simulink model "GNN_11612319_Ajay"  (R2021a)
settings: Solver=VariableStepAuto  StartTime=0.0  StopTime=1.0  RelTol=1e-8  AbsTol=1e-8
InitFcn:
  | I=eye(2);
  | k=10;
undefined symbols (not defined in the file): m
libraries: neural x1
settings Model: Creator=Mannaiyar  LastModifiedBy=Mannaiyar

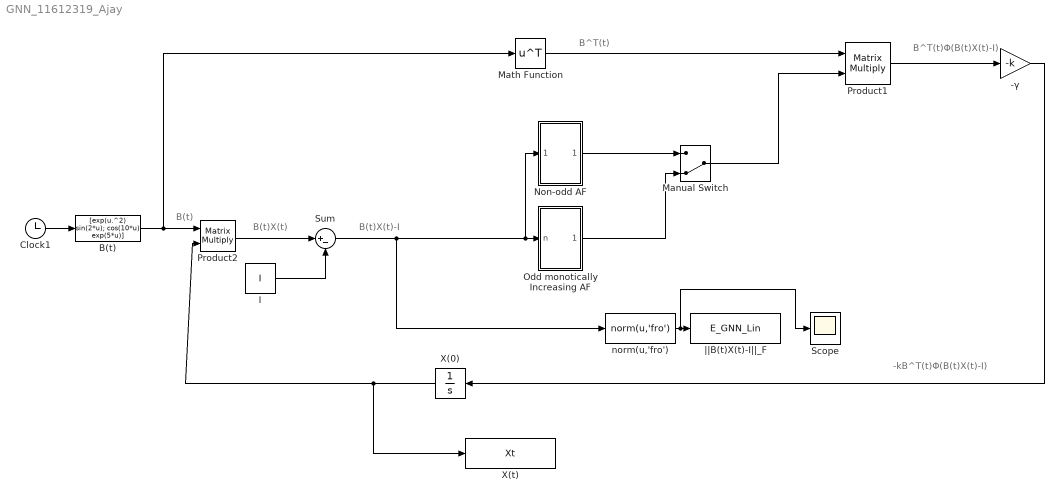
== system GNN_11612319_Ajay ==
  note: B(t)X(t)-I
  note: B(t)X(t)
  note: B(t)
  note: -kB^T(t)Φ(B(t)X(t)-I)
  note: B^T(t)
  note: B^T(t)Φ(B(t)X(t)-I)
  -γ : Gain  Gain=-k
  B(t) : MATLABFcn  MATLABFcn=[exp(u.^2) sin(2*u); cos(10*u) exp(5*u)]  Output1D=off
  Clock1 : Clock
  Manual Switch : ManualSwitch  CurrentSetting=0
  Math Function : Math  Operator=transpose  SignedPower=on  SaturateOnIntegerOverflow=on
  Non-odd AF : Subsystem
  Odd monotically Increasing AF : Subsystem
  Product1 : Product  Multiplication=Matrix(*)
  Product2 : Product  Multiplication=Matrix(*)
  Scope : Scope
  Sum : Sum  Inputs=|+-
  X(0) : Integrator
  X(t) : ToWorkspace  VariableName=Xt  SaveFormat=Timeseries  SampleTime=-1
  norm(u,'fro') : MATLABFcn  MATLABFcn=norm(u,'fro')  Output1D=off
  ||B(t)X(t)-I||_F : ToWorkspace  VariableName=E_GNN_Lin  SaveFormat=Timeseries  SampleTime=-1
  "Ι " : Constant  Value=I  VectorParams1D=off
  wires:
  Manual Switch/1 -> Product1/2
  Sum/1 -> norm(u,'fro')/1, Non-odd AF/1(In1), Odd monotically Increasing AF/1(n)
  Odd monotically Increasing AF/1(Out1) -> Manual Switch/2
  Math Function/1 -> Product1/1
  Clock1/1 -> B(t)/1
  B(t)/1 -> Math Function/1, Product2/1
  Non-odd AF/1(Out1) -> Manual Switch/1
  X(0)/1 -> X(t)/1, Product2/2
  Product2/1 -> Sum/1
  "Ι "/1 -> Sum/2
  -γ/1 -> X(0)/1
  norm(u,'fro')/1 -> Scope/1, ||B(t)X(t)-I||_F/1
  Product1/1 -> -γ/1

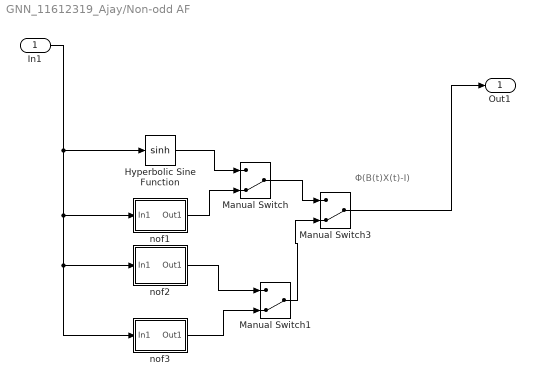
== system GNN_11612319_Ajay/Non-odd AF ==
  note: Φ(B(t)X(t)-I)
  In1 : Inport
  Hyperbolic Sine Function : Trigonometry  Operator=sinh
  Manual Switch : ManualSwitch  CurrentSetting=0
  Manual Switch1 : ManualSwitch  CurrentSetting=0
  Manual Switch3 : ManualSwitch  CurrentSetting=0
  "nof1 " : Subsystem
  nof2 : Subsystem
  nof3 : Subsystem
  Out1 : Outport
  wires:
  Hyperbolic Sine Function/1 -> Manual Switch/1
  nof2/1(Out1) -> Manual Switch1/1
  In1/1 -> nof3/1(In1), nof2/1(In1), "nof1 "/1(In1), Hyperbolic Sine Function/1
  "nof1 "/1(Out1) -> Manual Switch/2
  Manual Switch/1 -> Manual Switch3/1
  Manual Switch1/1 -> Manual Switch3/2
  nof3/1(Out1) -> Manual Switch1/2
  Manual Switch3/1 -> Out1/1

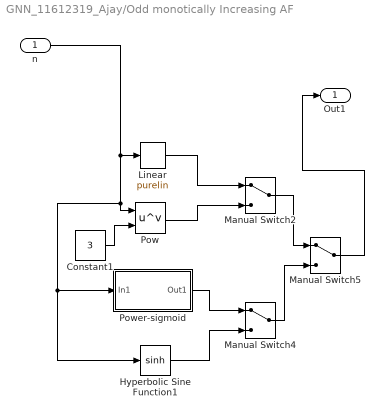
== system GNN_11612319_Ajay/Odd monotically Increasing AF ==
  n : Inport
  Constant1 : Constant  Value=3
  Hyperbolic Sine Function1 : Trigonometry  Operator=sinh
  Linear : neural/Transfer Functions/purelin
  Manual Switch2 : ManualSwitch
  Manual Switch4 : ManualSwitch
  Manual Switch5 : ManualSwitch
  Pow : Math  Operator=pow  SignedPower=on  SaturateOnIntegerOverflow=on
  "Power-sigmoid " : Subsystem
  Out1 : Outport
  wires:
  Linear/1 -> Manual Switch2/1
  Hyperbolic Sine Function1/1 -> Manual Switch4/2
  Constant1/1 -> Pow/2
  Manual Switch2/1 -> Manual Switch5/1
  n/1 -> Hyperbolic Sine Function1/1, "Power-sigmoid "/1(In1), Pow/1, Linear/1
  "Power-sigmoid "/1(Out1) -> Manual Switch4/1
  Manual Switch4/1 -> Manual Switch5/2
  Pow/1 -> Manual Switch2/2
  Manual Switch5/1 -> Out1/1

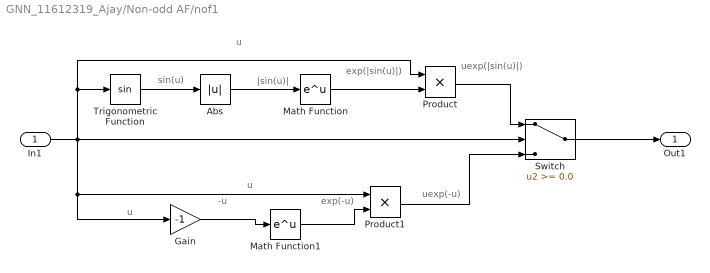
== system GNN_11612319_Ajay/Non-odd AF/nof1  ==
  note: uexp(-u)
  note: exp(-u)
  note: -u
  note: u
  note: u
  note: u
  note: exp(|sin(u)|)
  note: |sin(u)|
  note: sin(u)
  note: uexp(|sin(u)|)
  In1 : Inport
  Abs : Abs
  Gain : Gain  Gain=-1
  Math Function : Math  SignedPower=on  SaturateOnIntegerOverflow=on
  Math Function1 : Math  SignedPower=on  SaturateOnIntegerOverflow=on
  Product : Product
  Product1 : Product
  Switch : Switch  Threshold=0.0
  Trigonometric Function : Trigonometry
  Out1 : Outport
  wires:
  Switch/1 -> Out1/1
  In1/1 -> Gain/1, Product1/1, Product/1, Trigonometric Function/1, Switch/2
  Trigonometric Function/1 -> Abs/1
  Abs/1 -> Math Function/1
  Product/1 -> Switch/1
  Product1/1 -> Switch/3
  Math Function1/1 -> Product1/2
  Gain/1 -> Math Function1/1
  Math Function/1 -> Product/2

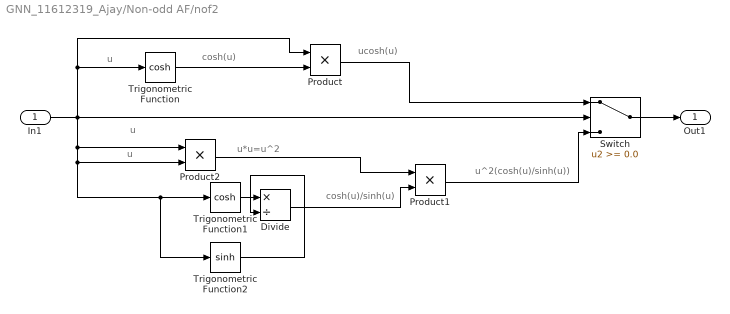
== system GNN_11612319_Ajay/Non-odd AF/nof2 ==
  note: u^2(cosh(u)/sinh(u))
  note: cosh(u)/sinh(u)
  note: u*u=u^2
  note: u
  note: u
  note: ucosh(u)
  note: cosh(u)
  note: u
  In1 : Inport
  Divide : Product  Inputs=*/
  Product : Product
  Product1 : Product
  Product2 : Product
  Switch : Switch  Threshold=0.0
  Trigonometric Function : Trigonometry  Operator=cosh
  Trigonometric Function1 : Trigonometry  Operator=cosh
  Trigonometric Function2 : Trigonometry  Operator=sinh
  Out1 : Outport
  wires:
  Switch/1 -> Out1/1
  In1/1 -> Product2/1, Trigonometric Function2/1, Trigonometric Function1/1, Product2/2, Product/1, Trigonometric Function/1, Switch/2
  Product/1 -> Switch/1
  Product1/1 -> Switch/3
  Divide/1 -> Product1/2
  Trigonometric Function/1 -> Product/2
  Product2/1 -> Product1/1
  Trigonometric Function1/1 -> Divide/1
  Trigonometric Function2/1 -> Divide/2

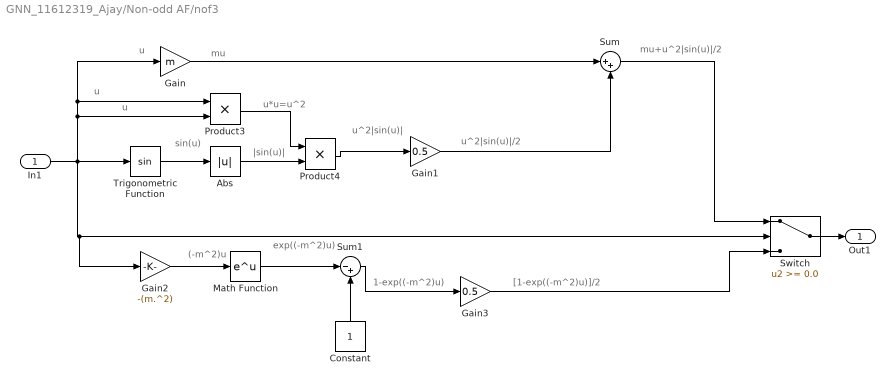
== system GNN_11612319_Ajay/Non-odd AF/nof3 ==
  note: exp((-m^2)u)
  note: (-m^2)u
  note: mu+u^2|sin(u)|/2
  note: u^2|sin(u)|/2
  note: u^2|sin(u)|
  note: |sin(u)|
  note: sin(u)
  note: u*u=u^2
  note: u
  note: u
  note: mu
  note: u
  note: 1-exp((-m^2)u)
  note: [1-exp((-m^2)u)]/2
  In1 : Inport
  Abs : Abs
  Constant : Constant
  Gain : Gain  Gain=m
  Gain1 : Gain  Gain=0.5
  Gain2 : Gain  Gain=-(m.^2)
  Gain3 : Gain  Gain=0.5
  Math Function : Math  SignedPower=on  SaturateOnIntegerOverflow=on
  Product3 : Product
  Product4 : Product
  Sum : Sum  Inputs=|++
  Sum1 : Sum  Inputs=|-+
  Switch : Switch  Threshold=0.0
  Trigonometric Function : Trigonometry
  Out1 : Outport
  wires:
  Switch/1 -> Out1/1
  In1/1 -> Trigonometric Function/1, Gain2/1, Switch/2, Product3/2, Product3/1, Gain/1
  Trigonometric Function/1 -> Abs/1
  Abs/1 -> Product4/2
  Product3/1 -> Product4/1
  Product4/1 -> Gain1/1
  Gain1/1 -> Sum/2
  Gain/1 -> Sum/1
  Sum/1 -> Switch/1
  Gain2/1 -> Math Function/1
  Math Function/1 -> Sum1/1
  Constant/1 -> Sum1/2
  Sum1/1 -> Gain3/1
  Gain3/1 -> Switch/3

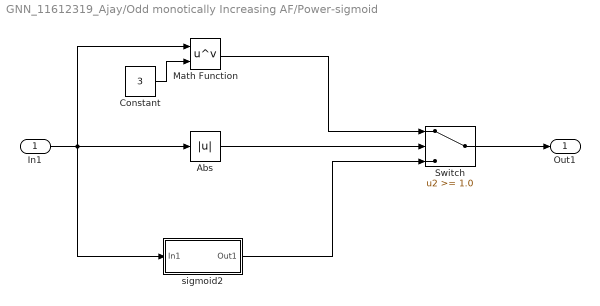
== system GNN_11612319_Ajay/Odd monotically Increasing AF/Power-sigmoid  ==
  In1 : Inport
  Abs : Abs
  Constant : Constant  Value=3
  Math Function : Math  Operator=pow  SignedPower=on  SaturateOnIntegerOverflow=on
  Switch : Switch  Threshold=1.0
  "sigmoid2 " : Subsystem
  Out1 : Outport
  wires:
  Switch/1 -> Out1/1
  Abs/1 -> Switch/2
  "sigmoid2 "/1(Out1) -> Switch/3
  Constant/1 -> Math Function/2
  Math Function/1 -> Switch/1
  In1/1 -> "sigmoid2 "/1(In1), Math Function/1, Abs/1

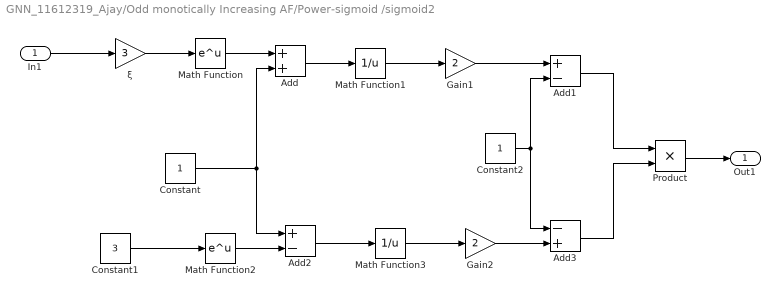
== system GNN_11612319_Ajay/Odd monotically Increasing AF/Power-sigmoid /sigmoid2  ==
  In1 : Inport
  Add : Sum
  Add1 : Sum  Inputs=+-
  Add2 : Sum  Inputs=+-
  Add3 : Sum  Inputs=-+
  Constant : Constant
  Constant1 : Constant  Value=3
  Constant2 : Constant
  Gain1 : Gain  Gain=2
  Gain2 : Gain  Gain=2
  Math Function : Math  SignedPower=on  SaturateOnIntegerOverflow=on
  Math Function1 : Math  Operator=reciprocal  SignedPower=on  SaturateOnIntegerOverflow=on
  Math Function2 : Math  SignedPower=on  SaturateOnIntegerOverflow=on
  Math Function3 : Math  Operator=reciprocal  SignedPower=on  SaturateOnIntegerOverflow=on
  Product : Product  RndMeth=Zero
  ξ : Gain  Gain=3
  Out1 : Outport
  wires:
  ξ/1 -> Math Function/1
  In1/1 -> ξ/1
  Math Function1/1 -> Gain1/1
  Gain1/1 -> Add1/1
  Product/1 -> Out1/1
  Add1/1 -> Product/1
  Math Function/1 -> Add/1
  Add/1 -> Math Function1/1
  Constant1/1 -> Math Function2/1
  Math Function2/1 -> Add2/2
  Constant/1 -> Add2/1, Add/2
  Add2/1 -> Math Function3/1
  Math Function3/1 -> Gain2/1
  Constant2/1 -> Add3/1, Add1/2
  Gain2/1 -> Add3/2
  Add3/1 -> Product/2
